simulink model "CH06_2"  (R2019a)
settings: Solver=VariableStepAuto  StartTime=0.0  StopTime=10.0  RelTol=1e-3
settings Model: Creator=吳俊逸  LastModifiedBy=吳俊逸

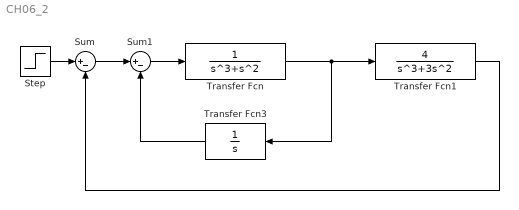
== system CH06_2 ==
  Step : Step  SampleTime=0
  Sum : Sum  Inputs=|+-
  Sum1 : Sum  Inputs=|+-
  Transfer Fcn : TransferFcn  Denominator=[1 1 0 0]
  Transfer Fcn1 : TransferFcn  Numerator=[4]  Denominator=[1 3 0 0]
  Transfer Fcn3 : TransferFcn  Denominator=[1 0]
  wires:
  Step/1 -> Sum/1
  Sum/1 -> Sum1/1
  Sum1/1 -> Transfer Fcn/1
  Transfer Fcn3/1 -> Sum1/2
  Transfer Fcn/1 -> Transfer Fcn3/1, Transfer Fcn1/1
  Transfer Fcn1/1 -> Sum/2
